simulink model "KF_3_gdl"  (R2020b)
settings: Solver=FixedStepAuto  StartTime=0.0  StopTime=1000  FixedStep=0.02  RelTol=1e-3
values from neighbouring files (symbols this model uses):
  b_x = -0.3    [init_3_gdl_AHRS_fb.m]    (also in init_3gdl.m = -0.03)
  b_y = 0.2    [init_3_gdl_AHRS_fb.m]    (also in init_3gdl.m = 0.02)
  b_z = 0.5    [init_3_gdl_AHRS_fb.m]    (also in init_3gdl.m = 0.05)
  BARO_cov = single(1.7)/2    [init_1gdl.m]    (also in init_3_gdl_AHRS_fb.m = single(1.7)/5; init_3gdl.m; init_dati_veri.m = single(1.7)/5)
  filter_pos = tf(1,[1 1])    [init_1gdl.m]    (also in init_3_gdl_AHRS_fb.m; init_3gdl.m; init_dati_veri.m)
  filter_pos_Z = tf(1,[0.5 1])    [init_3_gdl_AHRS_fb.m]    (also in init_3gdl.m; init_dati_veri.m)
  GPS_cov = single([1*2, 1])/2    [init_1gdl.m]    (also in init_3_gdl_AHRS_fb.m = single([0.1*50, 0.1*50, 200*5, 200*5, 0.36])/2; init_3gdl.m = single([1*2, 1*2, 1, 1, 0.36])/2; init_dati_veri.m = single([0.1, 0.1, 200*5, 200*5, 0.36])/2)
  IMU_cov = single(15*0.07)/2    [init_1gdl.m]    (also in init_3_gdl_AHRS_fb.m = single([15*[0.07*50, 0.07*50] 15*50*0.09])/2; init_3gdl.m = single([15*[0.07, 0.07] 10*0.09])/2; init_dati_veri.m = single([15*[0.07*5, 0.07*5] 15*50*0.09])/2)
  Q = single(diag([1e-2, 1e-6, 1e-4, 1e-12]))*2    [init_1gdl.m]    (also in init_3_gdl_AHRS_fb.m = single(diag([px,vx,ax,py,vy,ay,pz,vz,az,bx,by,bz]))*2; init_3gdl.m = single(diag([px,vx,ax,py,vy,ay,pz,vz,az,bx,by,bz]))*2; init_dati_veri.m = single(diag([px,vx,ax,py,vy,ay,pz,vz,az,bx,by,bz]))*2)
  Q_old = single(diag([1e-8, 1e-1, 1e-2, 1e-8, 1e-1, 1e-2, 1e-5, 1e-4, 0.010]))*2    [init_1gdl.m]    (also in init_3_gdl_AHRS_fb.m; init_3gdl.m; init_dati_veri.m)
  T_50 = 1/50    (= 0.02)    [init_1gdl.m]    (also in init_3_gdl_AHRS_fb.m; init_3gdl.m; init_dati_veri.m)
  var_p_x = 2    [init_3_gdl_AHRS_fb.m]    (also in init_3gdl.m = 1; init_dati_veri.m)
  var_p_y = 2    [init_3_gdl_AHRS_fb.m]    (also in init_3gdl.m = 1; init_dati_veri.m)
  var_p_z = 0.30    (= 0.3)    [init_3_gdl_AHRS_fb.m]    (also in init_3gdl.m = 0.15; init_dati_veri.m)
  var_v_x = 0.60    (= 0.6)    [init_3_gdl_AHRS_fb.m]    (also in init_3gdl.m = 0.3; init_dati_veri.m)
  var_v_y = 0.32    [init_3_gdl_AHRS_fb.m]    (also in init_3gdl.m = 0.16; init_dati_veri.m)
  var_v_z = 0.60    (= 0.6)    [init_3_gdl_AHRS_fb.m]    (also in init_3gdl.m = 0.3; init_dati_veri.m)
undefined symbols (not defined in the file or in its folder): DiscIntNeverNeededParam
libraries: cstblocks x12, simulink x9
settings Model: Creator=chiara-s  LastModifiedBy=chiara-s

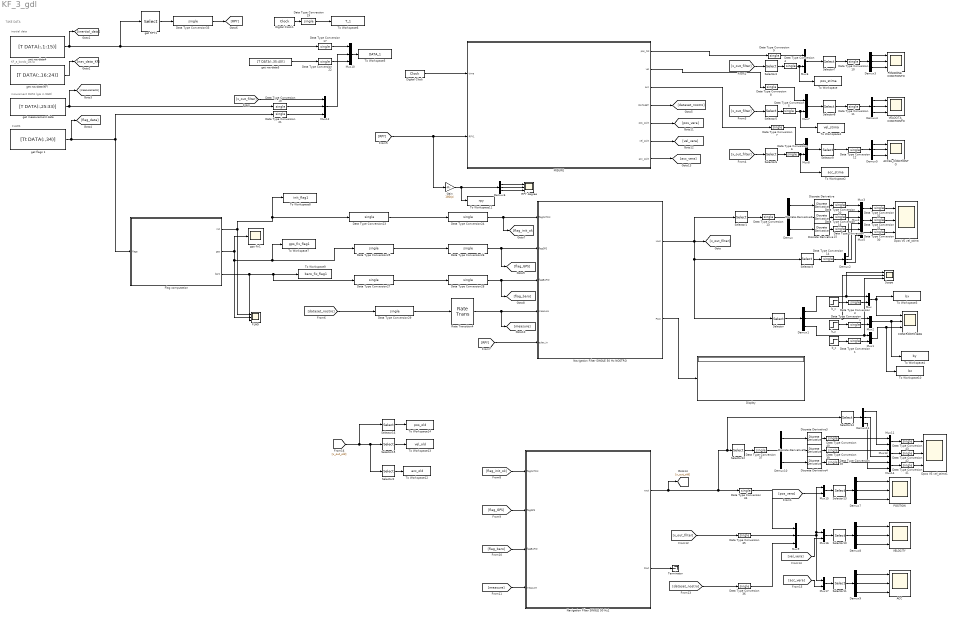
== system KF_3_gdl ==
  note: misurement DATA (già in NED)
  note: TAKE DATA
  note: inertial data
  note: KF_a_bordo_DATA
  note: FLAGS
  ACC : Scope  NumInputPorts=3
  ACCEL_CONFRONTO : Scope  NumInputPorts=3
  CONFRONTO BIAS : Scope  NumInputPorts=3
  Data Type Conversion{1..43} (43 alike) : DataTypeConversion  OutDataTypeStr=single
  Demux{,1..6,10..11} (9 alike) : Demux  Outputs=3
  Demux7 : Demux  Outputs=[4 4 4]
  Demux8 : Demux  Outputs=[4 4 4]
  Demux9 : Demux  Outputs=[4 4 4]
  Digital Clock : DigitalClock  SampleTime=0.02
  Digital Clock1 : DigitalClock  SampleTime=0.02
  Discrete Derivative{,1..5} (6 alike) : simulink/Discrete/Discrete Derivative  gainval=1.0  ICPrevScaledInput=0.0  OutMin=[]  OutMax=[]  OutDataType=fixdt(1, 16)  OutScaling=2^-10  DoSatur=off
  Display : Display
  Dpos VS vel_stima : Scope  NumInputPorts=3
  Dpos VS vel_stima1 : Scope  NumInputPorts=3
  FLAG : Scope  NumInputPorts=3
  Flag computation : MATLAB Function  TreatAsAtomicUnit=on
  Gain : Gain  Gain=180/pi
  MISURE : Subsystem
  Mux{,1..8,11,13..17} (15 alike) : Mux  Inputs=2
  Mux10 : Mux  Inputs=3
  Mux12 : Mux  Inputs=3
  Mux9 : Mux  Inputs=3
  Navigation Filter SINGLE 50 Hz NOSTRO : MATLAB Function  TreatAsAtomicUnit=on  mask{Q=Q, GPS_cov=GPS_cov, IMU_cov=IMU_cov, BARO_cov=BARO_cov}
      mask prompts: Q "Q matrix"; GPS_cov "R matrix - GPS covariance [px py vx vy vz]"; IMU_cov "R matrix - IMU covariance [ax ay az]"; BARO_cov "R matrix - BARO covariance"
  Navigation Filter SINGLE 50 Hz1 : MATLAB Function  TreatAsAtomicUnit=on  mask{Q=Q_old, GPS_cov=GPS_cov, IMU_cov=IMU_cov, BARO_cov=BARO_cov}
      mask prompts: Q "Q matrix"; GPS_cov "R matrix - GPS covariance [px py vx vy vz]"; IMU_cov "R matrix - IMU covariance [ax ay az]"; BARO_cov "R matrix - BARO covariance"
  POSITION : Scope  NumInputPorts=3
  POSIZIONE_CONFRONTO : Scope  NumInputPorts=3
  RPY degree : Scope  NumInputPorts=3
  Rate Transition4 : RateTransition  OutPortSampleTime=1/50
  Scope : Scope  NumInputPorts=3
  Selector : Selector  InputPortWidth=12  IndexOptions=Index vector (dialog)  Indices=[10 11 12]  OutputSizes=1
  Selector1 : Selector  InputPortWidth=12  IndexOptions=Index vector (dialog)  Indices=[1 4 7]  OutputSizes=1
  Selector10 : Selector  InputPortWidth=30+3  IndexOptions=Index vector (dialog)  Indices=[2 11 23 31 5 14 26 32 8 17 29 33]  OutputSizes=1
  Selector11 : Selector  InputPortWidth=30+3  IndexOptions=Index vector (dialog)  Indices=[3 12 24 31 6 15 27 32 9 18 30 33]  OutputSizes=1
  Selector12 : Selector  InputPortWidth=9  IndexOptions=Index vector (dialog)  Indices=[1 4 7]  OutputSizes=1
  Selector13 : Selector  InputPortWidth=30+3  IndexOptions=Index vector (dialog)  Indices=[1 10 22 31 4 13 25 32 7 16 28 33]  OutputSizes=1
  Selector14 : Selector  InputPortWidth=9  IndexOptions=Index vector (dialog)  Indices=[2 5 8]  OutputSizes=1
  Selector15 : Selector  InputPortWidth=9  IndexOptions=Index vector (dialog)  Indices=[2 5 8]  OutputSizes=1
  Selector16 : Selector  InputPortWidth=9  IndexOptions=Index vector (dialog)  Indices=[1 4 7]  OutputSizes=1
  Selector2 : Selector  InputPortWidth=9  IndexOptions=Index vector (dialog)  Indices=[3 6 9]  OutputSizes=1
  Selector3 : Selector  InputPortWidth=12  IndexOptions=Index vector (dialog)  Indices=[2 5 8]  OutputSizes=1
  Selector4 : Selector  InputPortWidth=12  IndexOptions=Index vector (dialog)  Indices=[1 4 7]  OutputSizes=1
  Selector5 : Selector  InputPortWidth=12  IndexOptions=Index vector (dialog)  Indices=[2 5 8]  OutputSizes=1
  Selector6 : Selector  InputPortWidth=12  IndexOptions=Index vector (dialog)  Indices=[3 6 9]  OutputSizes=1
  Selector7 : Selector  InputPortWidth=9  IndexOptions=Index vector (dialog)  Indices=[1 2 7 3 4 8 5 6 9]  OutputSizes=1
  Selector8 : Selector  InputPortWidth=9  IndexOptions=Index vector (dialog)  Indices=[1 2 7 3 4 8 5 6 9]  OutputSizes=1
  Selector9 : Selector  InputPortWidth=9  IndexOptions=Index vector (dialog)  Indices=[1 2 7 3 4 8 5 6 9]  OutputSizes=1
  Terminator : Terminator
  To Workspace : ToWorkspace  VariableName=pos_stima  SaveFormat=Timeseries  SampleTime=-1
  To Workspace1 : ToWorkspace  VariableName=vel_stima  SaveFormat=Timeseries  SampleTime=-1
  To Workspace10 : ToWorkspace  VariableName=bz  SaveFormat=Timeseries  SampleTime=-1
  To Workspace11 : ToWorkspace  VariableName=rpy  SaveFormat=Timeseries  SampleTime=-1
  To Workspace12 : ToWorkspace  VariableName=acc_old  SaveFormat=Timeseries  SampleTime=-1
  To Workspace13 : ToWorkspace  VariableName=vel_old  SaveFormat=Timeseries  SampleTime=-1
  To Workspace14 : ToWorkspace  VariableName=pos_old  SaveFormat=Timeseries  SampleTime=-1
  To Workspace2 : ToWorkspace  VariableName=acc_stima  SaveFormat=Timeseries  SampleTime=-1
  To Workspace3 : ToWorkspace  VariableName=bx  SaveFormat=Timeseries  SampleTime=-1
  To Workspace4 : ToWorkspace  VariableName=by  SaveFormat=Timeseries  SampleTime=-1
  To Workspace5 : ToWorkspace  VariableName=DATA_1  SampleTime=-1
  To Workspace6 : ToWorkspace  VariableName=T_1  SampleTime=-1
  To Workspace7 : ToWorkspace  VariableName=gps_fix_flag1  SampleTime=-1
  To Workspace8 : ToWorkspace  VariableName=init_flag1  SampleTime=-1
  To Workspace9 : ToWorkspace  VariableName=baro_fix_flag1  SampleTime=-1
  VELOCITA_CONFRONTO : Scope  NumInputPorts=3
  VELOCITY : Scope  NumInputPorts=3
  b_x : Step  Time=0  After=b_x  SampleTime=T_50
  b_y : Step  Time=0  After=b_y  SampleTime=T_50
  b_z : Step  Time=0  After=b_z  SampleTime=T_50
  get RPY1 : Selector  InputPortWidth=15  IndexOptions=Index vector (dialog)  Indices=[2:4]  OutputSizes=1
  get flags 1 : FromWorkspace  VariableName=[Tt DATA(:,34)]  SampleTime=0.02  OutputAfterFinalValue=Holding final value
  "get measurement data " : FromWorkspace  VariableName=[T DATA(:,25:33)]  SampleTime=0.02  OutputAfterFinalValue=Holding final value
  get navdata(KF) : FromWorkspace  VariableName=[T DATA(:,16:24)]  SampleTime=0.02  OutputAfterFinalValue=Holding final value
  get navdata4 : FromWorkspace  VariableName=[T DATA(:,1:15)]  SampleTime=0.02  Interpolate=off  OutputAfterFinalValue=Holding final value
  get navdata5 : FromWorkspace  VariableName=[T DATA(:,35:40)]  SampleTime=0.02  Interpolate=off  OutputAfterFinalValue=Holding final value
  gps fix1 : Scope
  wires:
  Data Type Conversion19/1 -> To Workspace6/1
  Data Type Conversion25/1 -> Data Type Conversion26/1
  Data Type Conversion17/1 -> Mux10/1
  Data Type Conversion29/1 -> Rate Transition4/1
  [x_out_filter] -> Mux12/1
  Data Type Conversion28/1 -> [flag_baro], Navigation Filter SINGLE 50 Hz NOSTRO/3(flagBARO)
  Navigation Filter SINGLE 50 Hz NOSTRO/1(xout) -> Selector/1, Selector3/1, [x_out_filter], Selector1/1
  get navdata4/1 -> get RPY1/1, Data Type Conversion17/1, [inertial_data]
  Data Type Conversion18/1 -> Mux12/2
  Data Type Conversion24/1 -> [flag_init_ok], Navigation Filter SINGLE 50 Hz NOSTRO/1(flagINITOK)
  Mux12/1 -> Mux10/2
  Data Type Conversion22/1 -> Mux10/3
  Data Type Conversion27/1 -> Data Type Conversion28/1
  Flag computation/1(init) -> FLAG/1, To Workspace8/1, Data Type Conversion23/1
  Data Type Conversion21/1 -> Mux12/3
  get navdata5/1 -> Data Type Conversion22/1
  Digital Clock1/1 -> Data Type Conversion19/1
  Navigation Filter SINGLE 50 Hz NOSTRO/2(Pout) -> Display/1
  Data Type Conversion26/1 -> [flag_GPS], Navigation Filter SINGLE 50 Hz NOSTRO/2(flagGPS)
  get flags 1/1 -> [flag_data], Flag computation/1(flags), Data Type Conversion21/1
  Rate Transition4/1 -> [measure], Navigation Filter SINGLE 50 Hz NOSTRO/4(measure)
  Data Type Conversion23/1 -> Data Type Conversion24/1
  Flag computation/2(gps) -> To Workspace7/1, Data Type Conversion25/1, FLAG/2, gps fix1/1
  "get measurement data "/1 -> [measurements], Data Type Conversion18/1
  get navdata(KF)/1 -> [nav_data_KF]
  Flag computation/3(baro) -> FLAG/3, Data Type Conversion27/1, To Workspace9/1
  Mux10/1 -> To Workspace5/1
  Selector1/1 -> Data Type Conversion13/1
  Digital Clock/1 -> MISURE/1(time)
  [dataset_nostro] -> Data Type Conversion29/1
  MISURE/4(DATASET) -> [dataset_nostro]
  Selector/1 -> Demux1/1
  b_x/1 -> Data Type Conversion3/1
  Mux/1 -> CONFRONTO BIAS/1, To Workspace3/1
  Demux1/2 -> Scope/2, Mux2/1
  b_y/1 -> Data Type Conversion2/1
  Mux2/1 -> To Workspace4/1, CONFRONTO BIAS/2
  b_z/1 -> Data Type Conversion1/1
  Demux1/3 -> Scope/3, Mux1/1
  Mux1/1 -> To Workspace10/1, CONFRONTO BIAS/3
  Data Type Conversion1/1 -> Mux1/2
  Data Type Conversion2/1 -> Mux2/2
  Demux/1 -> Discrete Derivative/1
  Demux/2 -> Discrete Derivative2/1
  Demux/3 -> Discrete Derivative1/1
  Selector3/1 -> Data Type Conversion14/1
  Mux3/1 -> Data Type Conversion32/1
  Demux2/1 -> Mux3/2
  Mux4/1 -> Data Type Conversion31/1
  Demux2/2 -> Mux4/2
  Mux5/1 -> Data Type Conversion30/1
  Demux2/3 -> Mux5/2
  [x_out_filter] -> Selector4/1
  [x_out_filter] -> Selector5/1
  [x_out_filter] -> Selector6/1
  Selector4/1 -> Data Type Conversion4/1
  MISURE/1(pos_tot) -> Data Type Conversion9/1
  Mux6/1 -> Selector7/1
  Selector7/1 -> Data Type Conversion10/1
  Demux3/1 -> POSIZIONE_CONFRONTO/1
  Demux3/2 -> POSIZIONE_CONFRONTO/2
  Demux3/3 -> POSIZIONE_CONFRONTO/3
  Demux4/3 -> VELOCITA_CONFRONTO/3
  MISURE/2(vel) -> Data Type Conversion8/1
  Demux4/1 -> VELOCITA_CONFRONTO/1
  Mux7/1 -> Selector8/1
  Demux4/2 -> VELOCITA_CONFRONTO/2
  Selector5/1 -> Data Type Conversion5/1
  Demux5/3 -> ACCEL_CONFRONTO/3
  MISURE/3(acc) -> Data Type Conversion7/1
  Demux5/1 -> ACCEL_CONFRONTO/1
  Mux8/1 -> Selector9/1
  Demux5/2 -> ACCEL_CONFRONTO/2
  Selector6/1 -> Data Type Conversion6/1
  Data Type Conversion4/1 -> To Workspace/1, Mux6/2
  Data Type Conversion5/1 -> To Workspace1/1, Mux7/2
  Data Type Conversion6/1 -> To Workspace2/1, Mux8/2
  Data Type Conversion7/1 -> Mux8/1
  Data Type Conversion8/1 -> Mux7/1
  Data Type Conversion9/1 -> Mux6/1
  Data Type Conversion10/1 -> Demux3/1
  Selector8/1 -> Data Type Conversion11/1
  Data Type Conversion11/1 -> Demux4/1
  Data Type Conversion12/1 -> Demux5/1
  Selector9/1 -> Data Type Conversion12/1
  Data Type Conversion13/1 -> Demux/1
  Data Type Conversion14/1 -> Demux2/1
  Discrete Derivative1/1 -> Data Type Conversion15/1
  Data Type Conversion15/1 -> Mux5/1
  Discrete Derivative2/1 -> Data Type Conversion16/1
  Data Type Conversion16/1 -> Mux4/1
  Discrete Derivative/1 -> Data Type Conversion20/1
  Data Type Conversion20/1 -> Mux3/1
  Data Type Conversion30/1 -> Dpos VS vel_stima/3
  Data Type Conversion31/1 -> Dpos VS vel_stima/2
  Data Type Conversion32/1 -> Dpos VS vel_stima/1
  Data Type Conversion3/1 -> Mux/2
  Demux1/1 -> Scope/1, Mux/1
  get RPY1/1 -> Data Type Conversion33/1
  Data Type Conversion33/1 -> [RPY]
  [RPY] -> Gain/1, MISURE/2(RPY1)
  [RPY] -> Navigation Filter SINGLE 50 Hz NOSTRO/5(euler_in)
  Gain/1 -> To Workspace11/1, Demux6/1
  Demux6/1 -> RPY degree/1
  Demux6/2 -> RPY degree/2
  Demux6/3 -> RPY degree/3
  [flag_init_ok] -> Navigation Filter SINGLE 50 Hz1/1(flagINITOK)
  [flag_GPS] -> Navigation Filter SINGLE 50 Hz1/2(flagGPS)
  [flag_baro] -> Navigation Filter SINGLE 50 Hz1/3(flagBARO)
  [measure] -> Navigation Filter SINGLE 50 Hz1/4(measure)
  Navigation Filter SINGLE 50 Hz1/2(Pout) -> Terminator/1
  [x_out_filter] -> Data Type Conversion35/1
  [dataset_nostro] -> Data Type Conversion36/1
  Data Type Conversion34/1 -> Mux9/1
  Data Type Conversion35/1 -> Mux9/2
  Data Type Conversion36/1 -> Mux9/3
  Selector13/1 -> Demux7/1
  Demux7/1 -> POSITION/1
  Demux7/2 -> POSITION/2
  Demux7/3 -> POSITION/3
  Selector10/1 -> Demux8/1
  Selector11/1 -> Demux9/1
  Demux9/1 -> ACC/1
  Demux9/2 -> ACC/2
  Demux9/3 -> ACC/3
  Demux8/1 -> VELOCITY/1
  Demux8/2 -> VELOCITY/2
  Demux8/3 -> VELOCITY/3
  Discrete Derivative4/1 -> Data Type Conversion38/1
  Data Type Conversion37/1 -> Demux10/1
  Demux10/1 -> Discrete Derivative3/1
  Discrete Derivative3/1 -> Data Type Conversion40/1
  Discrete Derivative5/1 -> Data Type Conversion39/1
  Demux10/2 -> Discrete Derivative5/1
  Demux10/3 -> Discrete Derivative4/1
  Selector12/1 -> Data Type Conversion37/1
  Data Type Conversion40/1 -> Mux11/1
  Mux14/1 -> Data Type Conversion41/1
  Data Type Conversion39/1 -> Mux13/1
  Data Type Conversion41/1 -> Dpos VS vel_stima1/3
  Data Type Conversion38/1 -> Mux14/1
  Mux13/1 -> Data Type Conversion42/1
  Data Type Conversion42/1 -> Dpos VS vel_stima1/2
  Mux11/1 -> Data Type Conversion43/1
  Data Type Conversion43/1 -> Dpos VS vel_stima1/1
  Selector14/1 -> Demux11/1
  Demux11/1 -> Mux11/2
  Demux11/2 -> Mux13/2
  Demux11/3 -> Mux14/2
  Mux15/1 -> Selector13/1
  Mux16/1 -> Selector10/1
  Mux17/1 -> Selector11/1
  Mux9/1 -> Mux17/1, Mux15/1, Mux16/1
  [pos_vera] -> Mux15/2
  [vel_vera] -> Mux16/2
  MISURE/5(pos_pulit) -> [pos_vera]
  MISURE/7(acc_pulit) -> [acc_vera]
  MISURE/6(vel_pulit) -> [vel_vera]
  [acc_vera] -> Mux17/2
  Selector2/1 -> To Workspace12/1
  Navigation Filter SINGLE 50 Hz1/1(xout) -> [x_out_old], Selector14/1, Selector12/1, Data Type Conversion34/1
  [x_out_old] -> Selector16/1, Selector2/1, Selector15/1
  Selector16/1 -> To Workspace14/1
  Selector15/1 -> To Workspace13/1

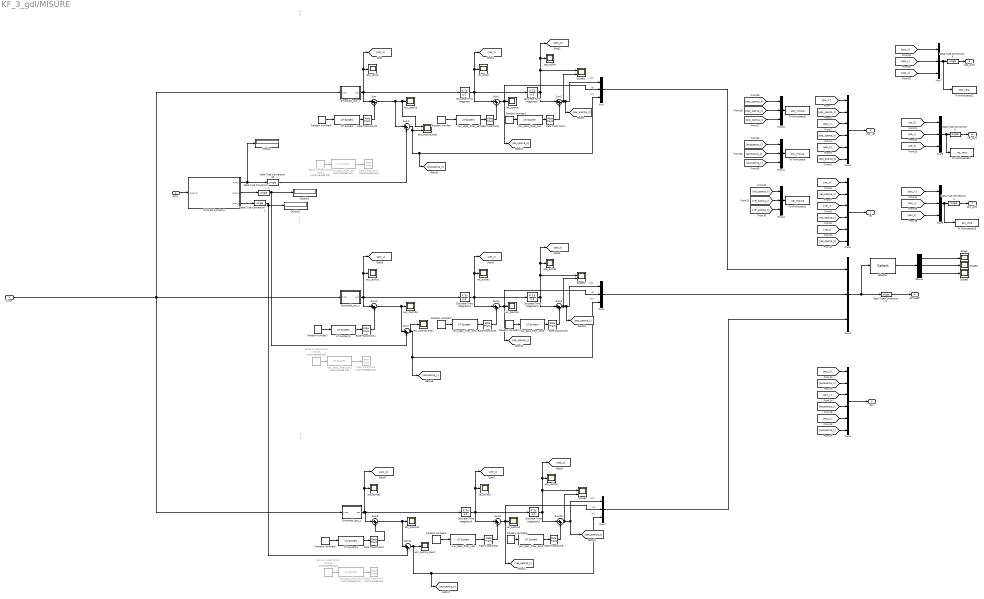
== system KF_3_gdl/MISURE ==
  note: X
  note: X
  note: acc
  note: vel
  note: pos
  note: y
  note: pos
  note: acc
  note: vel
  note: Y
  note: pos
  note: y
  note: acc
  note: vel
  note: Z
  time : Inport
  RPY1 : Inport  Port=2
  Band-Limited White Noise : simulink/Sources/Band-Limited White Noise  Commented=on  Cov=noise_gain  Ts=T_50  seed=[23341]
  Band-Limited White Noise1 : simulink/Sources/Band-Limited White Noise  Commented=on  Cov=noise_gain  Ts=T_50  seed=[23341]
  Band-Limited White Noise2 : simulink/Sources/Band-Limited White Noise  Commented=on  Cov=noise_gain  Ts=T_50  seed=[23341]
  Data Type Conversion{1..6,19} (7 alike) : DataTypeConversion  OutDataTypeStr=single
  Demux : Demux  Outputs=3
  Discrete-Time Integrator{,1..5} (6 alike) : DiscreteIntegrator  SampleTime=-1  ICPrevOutput=DiscIntNeverNeededParam  ICPrevScaledInput=DiscIntNeverNeededParam
  Display : Display
  Display1 : Display
  Display2 : Display
  LTI System : cstblocks/LTI System  sys=tf(1,[0.1 1])  IC=[]
  LTI System1 : cstblocks/LTI System  sys=tf(1,[0.1 1])  IC=[]
  LTI System2 : cstblocks/LTI System  sys=tf(1,[0.1 1])  IC=[]
  MATLAB Function1 : MATLAB Function  TreatAsAtomicUnit=on
  Mux{,1..3,7..12} (10 alike) : Mux  Inputs=3
  Mux4 : Mux  Inputs=6
  Mux5 : Mux  Inputs=6
  Mux6 : Mux  Inputs=6
  Random Number : RandomNumber  Variance=var_v_x  SampleTime=0.02
  Random Number1 : RandomNumber  Variance=var_p_x  Seed=1  SampleTime=0.02
  Random Number2 : RandomNumber  Variance=var_v_y  SampleTime=0.02
  Random Number3 : RandomNumber  Variance=var_p_y  Seed=1  SampleTime=0.02
  Random Number4 : RandomNumber  Variance=var_v_z  SampleTime=0.02
  Random Number5 : RandomNumber  Variance=var_p_z  Seed=1  SampleTime=0.02
  Random Number6 : RandomNumber  Variance=((0.07)/2)^2  SampleTime=0.02
  Random Number7 : RandomNumber  Variance=((0.07)/2)^2  SampleTime=0.02
  Random Number8 : RandomNumber  Variance=((0.07)/2)^2  SampleTime=0.02
  Rate Transition{1..2,5..6,8..12} (9 alike) : RateTransition  OutPortSampleTime=1/50
  Rate Transition3 : RateTransition  Commented=on  OutPortSampleTime=1/50
  Rate Transition4 : RateTransition  Commented=on  OutPortSampleTime=1/50
  Rate Transition7 : RateTransition  Commented=on  OutPortSampleTime=1/50
  Scope : Scope
  Scope1 : Scope  NumInputPorts=2
  Scope2 : Scope  NumInputPorts=2
  Scope3 : Scope  NumInputPorts=2
  Scope4 : Scope
  Scope5 : Scope
  Selector : Selector  InputPortWidth=9  IndexOptions=Index vector (dialog)  Indices=[1 4 7 2 5 8 3 6 9]  OutputSizes=1
  Sinusoidal_acc_x : MATLAB Function  TreatAsAtomicUnit=on
  Sinusoidal_acc_y : MATLAB Function  TreatAsAtomicUnit=on
  Sinusoidal_acc_z : MATLAB Function  TreatAsAtomicUnit=on
  Sum{,1..11} (12 alike) : Sum  Inputs=|++
  To Workspace : ToWorkspace  VariableName=acc_misura  SaveFormat=Timeseries  SampleTime=-1
  To Workspace1 : ToWorkspace  VariableName=vel_misura  SaveFormat=Timeseries  SampleTime=-1
  To Workspace11 : ToWorkspace  VariableName=pos_vera  SaveFormat=Timeseries  SampleTime=-1
  To Workspace12 : ToWorkspace  VariableName=vel_vera  SaveFormat=Timeseries  SampleTime=-1
  To Workspace13 : ToWorkspace  VariableName=acc_vera  SaveFormat=Timeseries  SampleTime=-1
  To Workspace2 : ToWorkspace  VariableName=pos_misura  SaveFormat=Timeseries  SampleTime=-1
  acc_pulita : Scope
  acc_pulita1 : Scope
  acc_pulita2 : Scope
  acc_sporca : Scope
  acc_sporca1 : Scope
  acc_sporca2 : Scope
  acc_sporca_bias : Scope  NumInputPorts=2
  acc_sporca_bias1 : Scope
  acc_sporca_bias2 : Scope
  low_pass_filter_acc : cstblocks/LTI System  Commented=on  sys=filter_acc  IC=[]
  low_pass_filter_acc1 : cstblocks/LTI System  Commented=on  sys=filter_acc  IC=[]
  low_pass_filter_acc2 : cstblocks/LTI System  Commented=on  sys=filter_acc  IC=[]
  low_pass_filter_pos : cstblocks/LTI System  sys=filter_pos*10  IC=[]
  low_pass_filter_pos1 : cstblocks/LTI System  sys=filter_pos*10  IC=[]
  low_pass_filter_pos2 : cstblocks/LTI System  sys=filter_pos_Z*10  IC=[]
  low_pass_filter_vel : cstblocks/LTI System  sys=filter_vel  IC=[]
  low_pass_filter_vel1 : cstblocks/LTI System  sys=filter_vel  IC=[]
  low_pass_filter_vel2 : cstblocks/LTI System  sys=filter_vel  IC=[]
  pos_pulita : Scope
  pos_pulita1 : Scope
  pos_pulita2 : Scope
  vel_pulita : Scope
  vel_pulita1 : Scope
  vel_pulita2 : Scope
  vel_sporca : Scope
  vel_sporca1 : Scope
  vel_sporca2 : Scope
  pos_tot : Outport
  vel : Outport  Port=2
  acc : Outport  Port=3
  DATASET : Outport  Port=4
  pos_pulit : Outport  Port=5
  vel_pulit : Outport  Port=6
  acc_pulit : Outport  Port=7
  wires:
  Sinusoidal_acc_x/1(acc) -> [acc_X], acc_pulita/1, Sum/1, Discrete-Time Integrator/1
  Mux/1 -> Mux3/1
  Discrete-Time Integrator/1 -> Sum1/1, Discrete-Time Integrator1/1, [vel_X], vel_pulita/1
  Discrete-Time Integrator1/1 -> Sum2/1, [pos_X], pos_pulita/1, Scope1/1
  Band-Limited White Noise/1 -> low_pass_filter_acc/1
  Sum/1 -> acc_sporca_bias/1, acc_sporca/1, Sum3/1
  low_pass_filter_acc/1 -> Rate Transition4/1
  low_pass_filter_vel/1 -> Rate Transition1/1
  Sum1/1 -> [vel_sporca_X], vel_sporca/1, Mux/2
  Sum2/1 -> Scope1/2, [pos_sporca_X], Mux/1
  Random Number/1 -> low_pass_filter_vel/1
  Random Number1/1 -> low_pass_filter_pos/1
  Sum3/1 -> [accsporca_X], Mux/3, acc_sporca_bias/2
  Sum4/1 -> Sum7/1, acc_sporca1/1
  Mux1/1 -> Mux3/2
  Sum7/1 -> [accsporca_y], Mux1/3, acc_sporca_bias1/1
  Random Number3/1 -> low_pass_filter_pos1/1
  Sum5/1 -> Mux1/2, vel_sporca1/1, [vel_sporca_y]
  Sum6/1 -> Scope2/2, [pos_sporca_y], Mux1/1
  low_pass_filter_acc1/1 -> Rate Transition3/1
  Discrete-Time Integrator3/1 -> Sum6/1, [pos_y], pos_pulita1/1, Scope2/1
  Band-Limited White Noise1/1 -> low_pass_filter_acc1/1
  Discrete-Time Integrator2/1 -> Sum5/1, Discrete-Time Integrator3/1, [vel_y], vel_pulita1/1
  low_pass_filter_vel1/1 -> Rate Transition5/1
  Sinusoidal_acc_y/1(acc) -> [acc_y], acc_pulita1/1, Sum4/1, Discrete-Time Integrator2/1
  Random Number2/1 -> low_pass_filter_vel1/1
  Sum8/1 -> Sum11/1, acc_sporca2/1
  low_pass_filter_vel2/1 -> Rate Transition8/1
  Mux2/1 -> Mux3/3
  Sum10/1 -> Scope3/2, [pos_sporca_z], Mux2/1
  Random Number4/1 -> low_pass_filter_vel2/1
  low_pass_filter_pos2/1 -> Rate Transition9/1
  Random Number5/1 -> low_pass_filter_pos2/1
  Sinusoidal_acc_z/1(acc) -> [acc_z], acc_pulita2/1, Sum8/1, Discrete-Time Integrator4/1
  Discrete-Time Integrator4/1 -> Sum9/1, Discrete-Time Integrator5/1, [vel_z], vel_pulita2/1
  Discrete-Time Integrator5/1 -> Sum10/1, [pos_z], pos_pulita2/1, Scope3/1
  time/1 -> Sinusoidal_acc_x/1(time), Sinusoidal_acc_z/1(time), Sinusoidal_acc_y/1(time)
  Sum9/1 -> Mux2/2, vel_sporca2/1, [vel_sporca_z]
  Band-Limited White Noise2/1 -> low_pass_filter_acc2/1
  low_pass_filter_acc2/1 -> Rate Transition7/1
  Sum11/1 -> acc_sporca_bias2/1, [accsporca_z], Mux2/3
  Mux3/1 -> Selector/1, Data Type Conversion3/1
  [pos_X] -> Mux4/1
  [pos_sporca_X] -> Mux4/2
  [pos_y] -> Mux4/3
  [pos_z] -> Mux4/5
  [pos_sporca_y] -> Mux4/4
  [pos_sporca_z] -> Mux4/6
  Mux4/1 -> pos_tot/1
  Mux5/1 -> vel/1
  [vel_X] -> Mux5/1
  [vel_sporca_X] -> Mux5/2
  [vel_y] -> Mux5/3
  [vel_sporca_y] -> Mux5/4
  [vel_sporca_z] -> Mux5/6
  [vel_z] -> Mux5/5
  [acc_z] -> Mux6/5
  [accsporca_y] -> Mux6/4
  [acc_y] -> Mux6/3
  [accsporca_X] -> Mux6/2
  [acc_X] -> Mux6/1
  Mux6/1 -> acc/1
  [accsporca_z] -> Mux6/6
  Data Type Conversion3/1 -> DATASET/1
  RPY1/1 -> MATLAB Function1/1(euler_in)
  MATLAB Function1/1(bias_x) -> Display/1, Data Type Conversion19/1
  MATLAB Function1/2(bias_y) -> Data Type Conversion1/1
  MATLAB Function1/3(bias_z) -> Data Type Conversion2/1
  Data Type Conversion19/1 -> Sum3/2
  Data Type Conversion1/1 -> Sum7/2, Display1/1
  Data Type Conversion2/1 -> Sum11/2, Display2/1
  Selector/1 -> Demux/1
  Demux/1 -> Scope/1
  Demux/2 -> Scope4/1
  Demux/3 -> Scope5/1
  Rate Transition1/1 -> Sum1/2
  low_pass_filter_pos/1 -> Rate Transition2/1
  Rate Transition2/1 -> Sum2/2
  Rate Transition5/1 -> Sum5/2
  Rate Transition6/1 -> Sum6/2
  low_pass_filter_pos1/1 -> Rate Transition6/1
  Rate Transition8/1 -> Sum9/2
  Rate Transition9/1 -> Sum10/2
  [pos_X] -> Mux7/1
  [pos_y] -> Mux7/2
  [pos_z] -> Mux7/3
  [vel_X] -> Mux8/1
  [vel_y] -> Mux8/2
  [vel_z] -> Mux8/3
  [acc_z] -> Mux9/3
  [acc_y] -> Mux9/2
  [acc_X] -> Mux9/1
  Mux9/1 -> To Workspace13/1, Data Type Conversion4/1
  Data Type Conversion4/1 -> acc_pulit/1
  Mux8/1 -> To Workspace12/1, Data Type Conversion5/1
  Data Type Conversion5/1 -> vel_pulit/1
  Mux7/1 -> To Workspace11/1, Data Type Conversion6/1
  Data Type Conversion6/1 -> pos_pulit/1
  LTI System/1 -> Rate Transition10/1
  Random Number6/1 -> LTI System/1
  Rate Transition10/1 -> Sum/2
  LTI System1/1 -> Rate Transition11/1
  Random Number7/1 -> LTI System1/1
  Rate Transition11/1 -> Sum4/2
  LTI System2/1 -> Rate Transition12/1
  Random Number8/1 -> LTI System2/1
  Rate Transition12/1 -> Sum8/2
  [pos_sporca_X] -> Mux10/1
  [pos_sporca_y] -> Mux10/2
  [pos_sporca_z] -> Mux10/3
  Mux10/1 -> To Workspace2/1
  Mux11/1 -> To Workspace/1
  [accsporca_X] -> Mux11/1
  [accsporca_y] -> Mux11/2
  [accsporca_z] -> Mux11/3
  Mux12/1 -> To Workspace1/1
  [vel_sporca_X] -> Mux12/1
  [vel_sporca_y] -> Mux12/2
  [vel_sporca_z] -> Mux12/3

== matlab function KF_3_gdl/MISURE/Sinusoidal_acc_x ==
  settings: updateMethod=DISCRETE  sampleTime=0.02
  data: time input; acc output
function acc = fcn(time)

t = time;

a = 0.02*sin(0.01*t);
b = (0.03)*sin(0.03*t + pi);
c = (0.04)*sin(0.04*t + pi/2);
if t >= 0 && t < 107 
    acc = 0;
else
    acc = a + b + c;
    acc = acc - 0.0061;
end

end

== matlab function KF_3_gdl/Flag computation ==
  data: flags input; init output; gps output; baro output
function [init,gps,baro] = fcn(flags)
%#codegen
%flags = init*100 + baro*10 + gps;

% centinaia: 
if flags > 50
    init = 1;
else
    init = 0;
end
%decine 
if flags-init*100 > 5
    baro = 1;
else
    baro = 0;
end
%unità
if flags-init*100-baro*10 > 0.5
    gps = 1;
else
    gps = 0;
end


% flags = 100 + 10 + 1;
% init 100
% init + gps 110
% init + gps + baro = 111
% init + baro = 101

== matlab function KF_3_gdl/Navigation Filter SINGLE 50 Hz NOSTRO ==
  data: flagINITOK input single size=1; flagGPS input single size=1; flagBARO input single size=1; xout output single size=12; measure input single size=9; Q parameter single size=[12,12]; GPS_cov parameter single size=5; BARO_cov parameter single size=1; IMU_cov parameter single size=3; Pout output single; euler_in input
function [xout,Pout] = GPS_BARO_KF_opt( flagINITOK, flagGPS, flagBARO, measure, Q, GPS_cov, BARO_cov, IMU_cov,euler_in)
coder.extrinsic('body2ned')
%% definition of variables
persistent P %covariance matrix 
persistent x %state vector
persistent filter_running
%filter matrices and constants
persistent A B 
persistent C_GPS_tot R_GPS_tot C_GPS_pos_vel R_GPS_pos_vel C_BARO R_BARO C_IMU R_IMU

if isempty(P)
   % esce qualcosa
%      P = single(0.1)*Q; % Q da cambiare (dimensioni e valori)
%      P(10,10) = 100;
%      P(11,11) = 100;
%      P(12,12) = 100;
% prove robustezza
       P = single(1)*eye(12); % Q da cambiare (dimensioni e valori)
       P(10,10) = 50;
       P(11,11) = 50;
       P(12,12) = 50;

    % Augmented State (pos, vel, acc, bias  -  3 gdl)
    x = single(zeros(12,1));
    
    filter_running = logical(false); %filter starts in OFF, must wait for flagINITOK to become true
    
    dt = single(0.02);
    %u  = 0;
    
    subM =    [1, dt,  0.5*dt^2;
               0,  1,        dt;
               0,  0,        1];
        
    A = [      subM, zeros(3,3), zeros(3,3), zeros(3,3);
         zeros(3,3),       subM, zeros(3,3), zeros(3,3);
         zeros(3,3), zeros(3,3),       subM, zeros(3,3);
         zeros(3,3), zeros(3,3), zeros(3,3),  eye(3,3)];
            
    
    % Augmented B
    B = single(eye(12,1));

    % Augmented Covariance state matrix (eps = bias accelerometer - body frame)
    % px|vx|ax|py|vy|ay|pz|vz|az|eps_x|eps_y|eps_z|
    % Q from init 

    % Covariance output matrix
    % GPS covariances = px|vx|py|vy|pz|
    % GPS_cov  = [0.03, 0.05, 0.016, 0.014, 0.36]; from init
    % IMU covariances = ax|ay|az|
    % IMU_cov  = 1000*[0.07, 0.07, 0.09];    from init
    % BARO_cov =  1.7; from init 

%   Rotation Matrix from body to navigation frame
    phi = euler_in(1);
    theta = euler_in(2);
    psi = euler_in(3);
    C = zeros(3,3,'single');
%     C = body2ned(phi,theta,psi);
    C = single(eye(3));

     %output matrices 
    %tutte le misure disponibili 
    C_GPS_tot = single([ 1 0 0  0 0 0  0 0 0       0          0         0;
                         0 1 0  0 0 0  0 0 0       0          0         0;
                         0 0 1  0 0 0  0 0 0   C(1,1)    C(1,2)    C(1,3);
                         0 0 0  1 0 0  0 0 0       0          0         0;
                         0 0 0  0 1 0  0 0 0       0          0         0;
                         0 0 0  0 0 1  0 0 0   C(2,1)    C(2,2)    C(2,3);
                         0 0 0  0 0 0  1 0 0       0          0         0;
                         0 0 0  0 0 0  0 0 1   C(3,1)    C(3,2)    C(3,3)]);                                                                                                                                                                                                                                                                                                                                                                                                                                                                                                                                                                                                                                                                                                                                                                                                                   ;
    
    R_GPS_tot = diag([GPS_cov(1),GPS_cov(3), IMU_cov(1),...
                      GPS_cov(2),GPS_cov(4), IMU_cov(2),...
                      BARO_cov,   IMU_cov(3)]);
    
    % vel GPS, pos GPS & IMU
    C_GPS_pos_vel = single([ 1 0 0  0 0 0  0 0 0        0          0         0;
                             0 1 0  0 0 0  0 0 0        0          0         0;
                             0 0 1  0 0 0  0 0 0    C(1,1)    C(1,2)    C(1,3);
                             0 0 0  1 0 0  0 0 0        0          0         0;
                             0 0 0  0 1 0  0 0 0        0          0         0;
                             0 0 0  0 0 1  0 0 0    C(2,1)    C(2,2)    C(2,3);
                             0 0 0  0 0 0  0 0 1   C(3,1)    C(3,2)    C(3,3)]);
                         
    R_GPS_pos_vel = diag([GPS_cov(1),GPS_cov(3), IMU_cov(1),...
                          GPS_cov(2),GPS_cov(4), IMU_cov(2),...
                          IMU_cov(3)]);
    % Baro & IMU
    C_BARO = single([0, 0, 1, 0, 0, 0, 0, 0, 0  C(1,1)    C(1,2)    C(1,3);
                     0, 0, 0, 0, 0, 1, 0, 0, 0  C(2,1)    C(2,2)    C(2,3);
                     0, 0, 0, 0, 0, 0, 1, 0, 0      0          0         0;         
                     0, 0, 0, 0, 0, 0, 0, 0, 1  C(3,1)    C(3,2)    C(3,3)]);
                 
    R_BARO = diag([IMU_cov(1),...
                   IMU_cov(2),...
                   BARO_cov, IMU_cov(3)]);
                 
    % solo IMU
    C_IMU = single([0, 0, 1, 0, 0, 0, 0, 0, 0  C(1,1)    C(1,2)    C(1,3);
                    0, 0, 0, 0, 0, 1, 0, 0, 0  C(2,1)    C(2,2)    C(2,3);
                    0, 0, 0, 0, 0, 0, 0, 0, 1  C(3,1)    C(3,2)    C(3,3)]);
                
    R_IMU = diag([IMU_cov(1),...
                  IMU_cov(2),...
                  IMU_cov(3)]);
    
end

%%Rotation Matrix from body to navigation frame
    phi = euler_in(1);
    theta = euler_in(2);
    psi = euler_in(3);
    %C = body2ned(phi,theta,psi);
    C = single(eye(3,3));
    
C_GPS_tot(3,10:12) = [C(1,1) , C(1,2), C(1,3)];
C_GPS_tot(6,10:12) = [C(2,1) , C(2,2), C(2,3)];
C_GPS_tot(8,10:12) = [C(3,1) , C(3,2), C(3,3)];


C_GPS_pos_vel(3,10:12) = [C(1,1) , C(1,2), C(1,3)];
C_GPS_pos_vel(6,10:12) = [C(2,1) , C(2,2), C(2,3)];
C_GPS_pos_vel(7,10:12) = [C(3,1) , C(3,2), C(3,3)];


C_BARO(1,10:12) = [C(1,1) , C(1,2), C(1,3)];
C_BARO(2,10:12) = [C(2,1) , C(2,2), C(2,3)];
C_BARO(4,10:12) = [C(3,1) , C(3,2), C(3,3)];


C_IMU(1,10:12) = [C(1,1) , C(1,2), C(1,3)];
C_IMU(2,10:12) = [C(2,1) , C(2,2), C(2,3)];
C_IMU(3,10:12) = [C(3,1) , C(3,2), C(3,3)];


% x 12x1
%% initialization 
if and(not(filter_running),flagINITOK),
    % if filter is not running and initialization can be performed 
    % => initialize state = measure
    % => notify filter is running
    x= [measure; 0; 0; 0];
    filter_running = true;
end


%% TODO: capire che senso ha mettere u = 0 sempre 
u  = single(0);


if filter_running, 
    %% select update type (removed fuse types with separate gps pos and vel flags)
    if(flagGPS && flagBARO)
        fuse = 1;
    elseif(flagGPS)
        fuse = 2;
    elseif(flagBARO)
        fuse = 7;
    else
        fuse = 8;
    end

    %% Prediction
    [x, P] = predict(A, B, x, u, Q, P);


    %% Update
    switch fuse
        case 1
            % all measurements
            y = [measure(1), measure(2), measure(3), measure(4), measure(5), ...
                 measure(6), measure(7), measure(9)]';
            [x, P] = update(A, C_GPS_tot, x, y, P, R_GPS_tot);
        case 2
            % measurements of: pos GPS, vel GPS, IMU
            y = [measure(1), measure(2), measure(3), measure(4), measure(5), ...
                 measure(6),  measure(9)]';
            [x, P] = update(A, C_GPS_pos_vel, x, y, P, R_GPS_pos_vel);
        case 7
            % measurements of: BARO, IMU
            y = [measure(3), measure(6), measure(7), measure(9)]';
            [x, P] = update(A, C_BARO, x, y, P, R_BARO);
        case 8
            y = [measure(3), measure(6), measure(9)]';
            [x, P] = update(A, C_IMU, x, y, P, R_IMU);
    end
end

xout = x;
Pout = P;
end

function [x, P] = predict(A, B, x, u, Q, P)
    x = A*x + B*u;
    P = A*P*A' + Q;
end

function [x, P] = update(A, C, x, y, P, R)
    K = P*C'*inv(R + C*P*C');       % al max 4x3 se tutti sensori attivi
    x = x + K*(y - C*x);
    P = (eye(12) - K*C)*P;
    %P = 0.5*(P + transpose(P)); secondo me ci va, non dovrebbe fare male
end

== matlab function KF_3_gdl/MISURE/Sinusoidal_acc_y ==
  settings: updateMethod=DISCRETE  sampleTime=0.02
  data: time input; acc output
function acc = fcn(time)

t = time;

a = 0.02*sin(0.01*t);
b = (0.05)*sin(0.07*t + pi);
c = (0.04)*sin(0.05*t + pi/2);
if t >= 0 && t < 107 
    acc = 0;
else
    acc = a + b + c;
    acc = acc - 0.0037;
end

end

== matlab function KF_3_gdl/MISURE/Sinusoidal_acc_z ==
  settings: updateMethod=DISCRETE  sampleTime=0.02
  data: time input; acc output
function acc = fcn(time)

t = time;

a = 0.02*sin(0.01*t);
b = (0.03)*sin(0.05*t + pi);
c = (0.04)*sin(0.03*t + pi/2);
if t >= 0 && t < 107 
    acc = 0;
else
    acc = a + b + c;
    acc = acc - 0.0018;
end

end

== matlab function KF_3_gdl/MISURE/MATLAB Function1 ==
  data: euler_in input; bias_x output; bias_y output; bias_z output; b_x parameter; b_y parameter; b_z parameter
function [bias_x,bias_y,bias_z] = add_bias(euler_in,b_x, b_y, b_z)
coder.extrinsic('body2ned');
C = zeros(3,3,'single');
phi = euler_in(1);
theta = euler_in(2);
psi = euler_in(3); 
%C = body2ned(phi,theta,psi);
C = eye(3,3);
bias_body = [b_x; b_y; b_z];
bias_ned = C*bias_body;
bias_x = bias_ned(1);
bias_y = bias_ned(2);
bias_z = bias_ned(3);

end

== matlab function KF_3_gdl/Navigation Filter SINGLE 50 Hz1 ==
  data: flagINITOK input single size=1; flagGPS input single size=1; flagBARO input single size=1; xout output single size=9; measure input single size=9; Q parameter single size=[9,9]; GPS_cov parameter single size=5; BARO_cov parameter single size=1; IMU_cov parameter single size=3; Pout output single
function [xout,Pout] = GPS_BARO_KF_opt( flagINITOK, flagGPS, flagBARO, measure, Q, GPS_cov, BARO_cov, IMU_cov)
%% definition of variables
persistent P %covariance matrix 
persistent x %state vector
persistent filter_running
%filter matrices and constants
persistent A B 
persistent C_GPS_tot R_GPS_tot C_GPS_pos_vel R_GPS_pos_vel C_BARO R_BARO C_IMU R_IMU

if isempty(P)
    P = single(0.1)*Q;
    %initialize state with first measure
    x = single(zeros(9,1));
    
    filter_running = logical(false); %filter starts in OFF, must wait for flagINITOK to become true
    %prepare constant matrices for future use
    dt = single(0.02); 
    %u  = 0;
    subM = [1, dt, 0.5*dt^2;
            0,  1,       dt;
            0,  0,        1];
    A = [subM,zeros(3,3),zeros(3,3);
         zeros(3,3), subM, zeros(3,3);
         zeros(3,3),zeros(3,3),subM];
    B = single(zeros(9,1));
    B(9) = 1; % TODO_:capire che senso ha .... se u= 0 sempre 

    % Covariance state matrix
    % px|vx|ax|py|vy|ay|pz|vz|az
    % Q from mask 

    % Covariance output matrix
    % GPS covariances = px|py|vx|vy|vz
    % GPS_cov  = [0.03, 0.05, 0.016, 0.014, 0.36]; from mask
    % IMU covariances = ax|ay|az
    %IMU_cov  = 1000*[0.07, 0.07, 0.09];    from amsk
    %BARO_cov =  1.7; from amsk 

    %output matrices 
    %tutte le misure disponibili 
    C_GPS_tot = single([ 1 0 0  0 0 0  0 0 0;
                         0 1 0  0 0 0  0 0 0;
                         0 0 1  0 0 0  0 0 0;
                         0 0 0  1 0 0  0 0 0;
                         0 0 0  0 1 0  0 0 0;
                         0 0 0  0 0 1  0 0 0;
                         0 0 0  0 0 0  1 0 0;
                         0 0 0  0 0 0  0 0 1]);
    R_GPS_tot = diag([GPS_cov(1),GPS_cov(3), IMU_cov(1),...
                      GPS_cov(2),GPS_cov(4), IMU_cov(2),...
                      BARO_cov,   IMU_cov(3)]);
    
    % vel GPS, pos GPS & IMU
    C_GPS_pos_vel = single([ 1 0 0  0 0 0  0 0 0;
                             0 1 0  0 0 0  0 0 0;
                             0 0 1  0 0 0  0 0 0;
                             0 0 0  1 0 0  0 0 0;
                             0 0 0  0 1 0  0 0 0;
                             0 0 0  0 0 1  0 0 0;
                             0 0 0  0 0 0  0 0 1]);
                         
    R_GPS_pos_vel = diag([GPS_cov(1),GPS_cov(3), IMU_cov(1),...
                          GPS_cov(2),GPS_cov(4), IMU_cov(2),...
                          IMU_cov(3)]);
    % Baro & IMU
    C_BARO = single([0, 0, 1, 0, 0, 0, 0, 0, 0;
                     0, 0, 0, 0, 0, 1, 0, 0, 0;
                     0, 0, 0, 0, 0, 0, 1, 0, 0         % MANCA ; ????
                     0, 0, 0, 0, 0, 0, 0, 0, 1]);
                 
    R_BARO = diag([IMU_cov(1),...
                   IMU_cov(2),...
                   BARO_cov, IMU_cov(3)]);
    % solo IMU
    C_IMU = single([0, 0, 1, 0, 0, 0, 0, 0, 0;
                    0, 0, 0, 0, 0, 1, 0, 0, 0;
                    0, 0, 0, 0, 0, 0, 0, 0, 1]);
                
    R_IMU = diag([IMU_cov(1),...
                  IMU_cov(2),...
                  IMU_cov(3)]);
    
end

%% initialization 
if and(not(filter_running),flagINITOK),
    % if filter is not running and initialization can be performed 
    % => initialize state = measure
    % => notify filter is running
    x= measure;
    filter_running = true;
end


%% TODO: capire che senso ha mettere u = 0 sempre 
u  = single(0);


if filter_running, 
    %% select update type (removed fuse types with separate gps pos and vel flags)
    if(flagGPS && flagBARO)
        fuse = 1;
    elseif(flagGPS)
        fuse = 2;
    elseif(flagBARO)
        fuse = 7;
    else
        fuse = 8;
    end

    %% Prediction
    [x, P] = predict(A, B, x, u, Q, P);


    %% Update
    switch fuse
        case 1
            % all measurements
            y = [measure(1), measure(2), measure(3), measure(4), measure(5), ...
                 measure(6), measure(7), measure(9)]';
            [x, P] = update(A, C_GPS_tot, x, y, P, R_GPS_tot);
        case 2
            % measurements of: pos GPS, vel GPS, IMU
            y = [measure(1), measure(2), measure(3), measure(4), measure(5), ...
                 measure(6),  measure(9)]';
            [x, P] = update(A, C_GPS_pos_vel, x, y, P, R_GPS_pos_vel);
        case 7
            % measurements of: BARO, IMU
            y = [measure(3), measure(6), measure(7), measure(9)]';
            [x, P] = update(A, C_BARO, x, y, P, R_BARO);
        case 8
            y = [measure(3), measure(6), measure(9)]';
            [x, P] = update(A, C_IMU, x, y, P, R_IMU);
    end
end

xout = x;
Pout = P;
end

function [x, P] = predict(A, B, x, u, Q, P)
    x = A*x + B*u;
    P = A*P*A' + Q;
end

function [x, P] = update(A, C, x, y, P, R)
    K = P*C'*inv(R + C*P*C');
    x = x + K*(y - C*x);
    P = (eye(9) - K*C)*P;
    %P = 0.5*(P + transpose(P)); secondo me ci va, non dovrebbe fare male
end
